simulink model "AutomotiveEMS_2017b"  (R2017b)
settings: Solver=VariableStepAuto  StartTime=0  StopTime=0.1  MaxStep=1e-4  RelTol=1e-3
values from neighbouring files (symbols this model uses):
  iceToAltRotRatio = 2.5    [AutomotiveEMSRoutine.m]    (also in ControlComparisonRoutine.m; Main.m)
  T_s = 1.0e-6    (= 1e-06)    [AutomotiveEMSRoutine.m]    (also in ControlComparisonRoutine.m; HybridMPPTRoutine.m; LundellAlternatorACRoutine.m; LundellAlternatorDCRoutine.m)
undefined symbols (not defined in the file or in its folder): alternator, sigbuilder_block
libraries: fl_lib x74, nesl_utility x72, elec_lib x35, powerlib_meascontrol x2
(part 1 of 2)
settings Model: Creator=gabrielrodrigues  LastModifiedBy=gabrielrodrigues
settings CodeAppCC: StateflowObjectComments=on
settings SimscapeCC: SimscapeNormalizeSystem=off

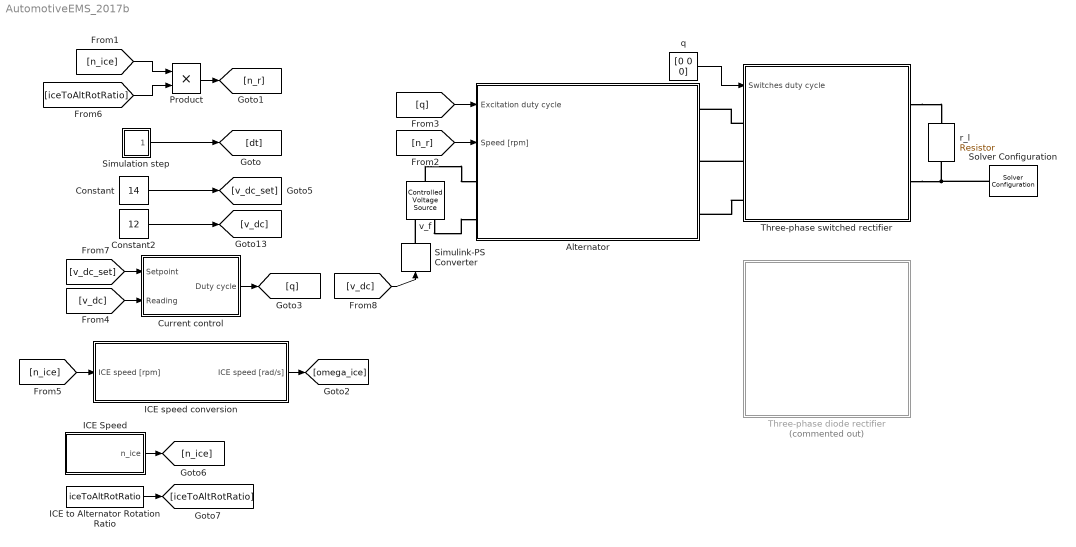
== system AutomotiveEMS_2017b ==
  Alternator : Subsystem
  Constant : Constant  Value=14
  Constant2 : Constant  Value=12
  Current control : Subsystem
  ICE Speed : Subsystem  Tag=STV Subsys  LoadFcn=sigbuilder_block('load');  StartFcn=sigbuilder_block('start');  StopFcn=sigbuilder_block('stop');  ClipboardFcn=sigbuilder_block('clipboard');  mask(Sigbuilder block){tuvar=[0:10]}
      mask help: Simulink:masks:SigbuilderBlock_MD
      mask init:
      | if ~strcmp(get_param(bdroot(gcbh),'SimulationStatus'),'stopped') tuvar = sigbuilder_block('maskInit'); end
      settings: CopyFcn=sigbuilder_block('copy');  DeleteFcn=sigbuilder_block('delete');  ModelCloseFcn=sigbuilder_block('modelClose');  PreSaveFcn=sigbuilder_block('preSave');  PauseFcn=sigbuilder_block('pause');  ContinueFcn=sigbuilder_block('continue');  NameChangeFcn=sigbuilder_block('namechange');  OpenFcn=sigbuilder_block('open',[433.5 195.75 558 399.75 ]);  CloseFcn=sigbuilder_block('close');
      mask Display: plot(0, 0, 100, 100,[2, 2, 32, 32, 2], [68, 8, 8, 68, 68],[32, 2], [38, 38], [32, 19, 2],[53, 60, 44], [32, 17, 17, 2],[16, 16, 31, 31]);txt = getActiveGroup(gcbh);text(2, 100, txt,'verticalAlignment', 'top');
  ICE speed conversion : Subsystem
  ICE to Alternator Rotation Ratio : Constant  Value=iceToAltRotRatio
  Product : Product
  Simulation step : Subsystem
  Simulink-PS Converter : nesl_utility/Simulink-PS Converter  PhysicalDomain=network_engine_domain  SubClassName=ps_input  LeftPortType=input  RightPortType=output  PseudoPeriodic=off  Frequencies=[]  NoiseDistribution=none  NoiseParameters=[]  Unit=1  AffineConversion=off  FilteringAndDerivatives=provide  SimscapeFilterOrder=1  InputFilterTimeConstant=0.001  UdotUserProvided=0
  Solver Configuration : nesl_utility/Solver Configuration  PhysicalDomain=network_engine_domain  SubClassName=solver  LeftPortType=input  RightPortType=generic  Tones=[]  Harmonics=[]  SimulateNoise=off  Profile=off  UseLocalSampling=off  EnableSwitchedLinearOptims=on  FrequencyDomain=off  UseCCode=off  RelTol=0.001  AbsTol=1e-06  MinStep=1e-09  ToWorkspace=off  RevertToSquareIcSolve=off  NumHomotopyIterations=100  PhasorMode=off  PhasorModeNumHarmonics=1  DoDC=off  ResidualTolerance=1e-09  UseLocalSolver=off  LocalSolverChoice=NE_BACKWARD_EULER_ADVANCER  LocalSolverSampleTime=0.001  DoFixedCost=off  MaxNonlinIter=3  MaxModeIter=2  LinearAlgebra=Sparse  EquationFormulation=NE_TIME_EF  DelaysMemoryBudget=1024  AutomaticFiltering=on  FilteringTimeConstant=0.001
  Three-phase diode rectifier : Subsystem  Commented=on
  Three-phase switched rectifier : Subsystem
  q : Constant  Value=[0 0 0]
  r_l : elec_lib/Passive Devices/Resistor  R=1e+3 Ohm  R_tol=5  enable_R_tol=0  tol_distribution=1  nSigma=4  enable_operating_limits=0  operating_limit_action=2  max_working_voltage=100 V  power_rating=1 W  enable_faults=0  fault_action=1  R_faulted=inf Ohm  enable_temporal_fault=0  t_fault=1 s  enable_behavioral_fault=0  max_permissible_current=1 A  t_fail_on_current=1 s  noise_mode=0  sample_time=1e-3 s  repeatability=1  auto_seed=3922919431  user_seed=0  Tdevice=25 degC  alpha=3.93e-3 1/K  Tmeas=25 degC  thermal_mass=100 J/K  power_derating_T1=70 degC  power_derating_T2=155 degC  operating_temperature_range_vec=[-50, 150] degC  temperature_specify=off  temperature_priority=High  temperature=298.15 K  temperature_nominal_specify=off  temperature_nominal_unit=K  temperature_nominal_value=1
  v_f : fl_lib/Electrical/Electrical Sources/Controlled Voltage Source
  wires:
  [iceToAltRotRatio] -> Product/2
  [n_ice] -> Product/1
  Product/1 -> [n_r]
  Simulation step/1(step) -> [dt]
  ICE speed conversion/1(ICE speed [rad/s]) -> [omega_ice]
  Constant/1 -> [v_dc_set]
  [n_ice] -> ICE speed conversion/1(ICE speed [rpm])
  ICE to Alternator Rotation Ratio/1 -> [iceToAltRotRatio]
  Constant2/1 -> [v_dc]
  ICE Speed/1(n_ice) -> [n_ice]
  [n_r] -> Alternator/2(Speed [rpm])
  [q] -> Alternator/1(Excitation duty cycle)
  [v_dc] -> Current control/2(Reading)
  [v_dc_set] -> Current control/1(Setpoint)
  Current control/1(Duty cycle) -> [q]
  [v_dc] -> Simulink-PS Converter/1
  q/1 -> Three-phase switched rectifier/1(Switches duty cycle)
  connections:
  Three-phase switched rectifier/RConn1 -- r_l/LConn1
  Three-phase switched rectifier/LConn2 -- Alternator/RConn2
  Three-phase switched rectifier/LConn3 -- Alternator/RConn3
  Three-phase switched rectifier/LConn1 -- Alternator/RConn1
  Solver Configuration/RConn1 -- Three-phase switched rectifier/RConn2 -- r_l/RConn1
  v_f/LConn1 -- Alternator/LConn1
  v_f/RConn2 -- Alternator/LConn2
  Simulink-PS Converter/RConn1 -- v_f/RConn1

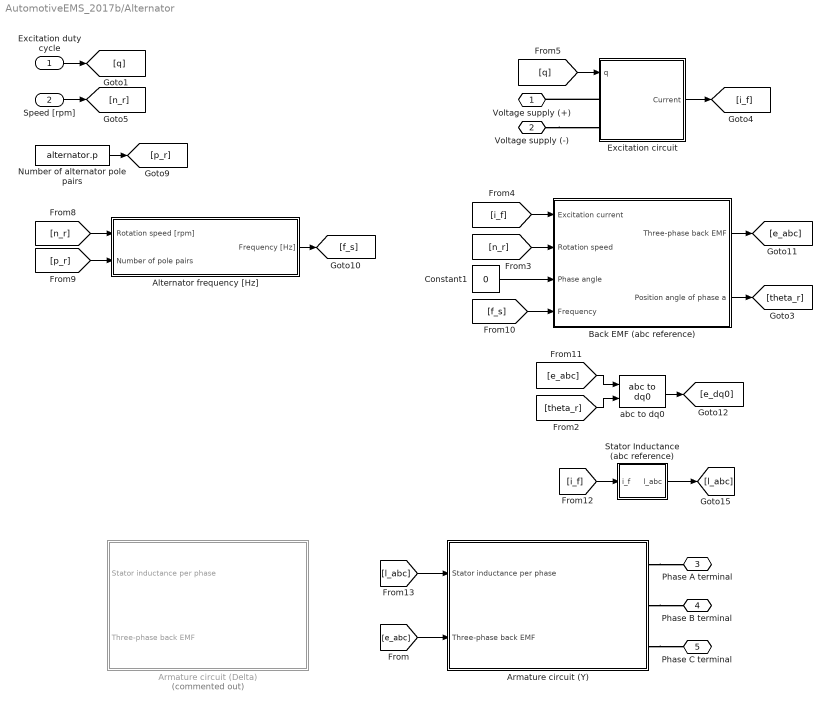
== system AutomotiveEMS_2017b/Alternator ==
  Excitation duty cycle : Inport
  Speed [rpm] : Inport  Port=2
  Alternator frequency [Hz] : Subsystem
  Armature circuit (Delta) : Subsystem  Commented=on
  Armature circuit (Y) : Subsystem
  Back EMF (abc reference) : Subsystem
  Constant1 : Constant  Value=0
  Excitation circuit : Subsystem
  Number of alternator pole pairs : Constant  Value=alternator.p
  Stator Inductance (abc reference) : Subsystem
  abc to dq0 : powerlib_meascontrol/Transformations/abc to dq0  Alignment=90 degrees behind phase A axis
  Voltage supply (+) : PMIOPort  Side=Left
  Voltage supply (-) : PMIOPort  Port=2  Side=Left
  Phase A terminal : PMIOPort  Port=3  Side=Right
  Phase B terminal : PMIOPort  Port=4  Side=Right
  Phase C terminal : PMIOPort  Port=5  Side=Right
  wires:
  Excitation circuit/1(Current) -> [i_f]
  Alternator frequency [Hz]/1(Frequency [Hz]) -> [f_s]
  Number of alternator pole pairs/1 -> [p_r]
  [n_r] -> Alternator frequency [Hz]/1(Rotation speed [rpm])
  [p_r] -> Alternator frequency [Hz]/2(Number of pole pairs)
  [i_f] -> Back EMF (abc reference)/1(Excitation current)
  [n_r] -> Back EMF (abc reference)/2(Rotation speed)
  Constant1/1 -> Back EMF (abc reference)/3(Phase angle)
  [f_s] -> Back EMF (abc reference)/4(Frequency)
  Back EMF (abc reference)/1(Three-phase back EMF) -> [e_abc]
  Back EMF (abc reference)/2(Position angle of phase a) -> [theta_r]
  [e_abc] -> abc to dq0/1
  [theta_r] -> abc to dq0/2
  abc to dq0/1 -> [e_dq0]
  [i_f] -> Stator Inductance (abc reference)/1(i_f)
  Stator Inductance (abc reference)/1(l_abc) -> [l_abc]
  [l_abc] -> Armature circuit (Y)/1(Stator inductance per phase)
  [e_abc] -> Armature circuit (Y)/2(Three-phase back EMF)
  Excitation duty cycle/1 -> [q]
  Speed [rpm]/1 -> [n_r]
  [q] -> Excitation circuit/1(q)
  connections:
  Armature circuit (Y)/RConn1 -- Phase A terminal/RConn1
  Armature circuit (Y)/RConn2 -- Phase B terminal/RConn1
  Armature circuit (Y)/RConn3 -- Phase C terminal/RConn1
  Excitation circuit/LConn1 -- Voltage supply (+)/RConn1
  Voltage supply (-)/RConn1 -- Excitation circuit/LConn2

== system AutomotiveEMS_2017b/Current control ==
  Setpoint : Inport
  Reading : Inport  Port=2
  Fcn : Fcn  Expr=u > 0
  Scope : Scope
  Sum : Sum  Inputs=+-
  Duty cycle : Outport
  wires:
  Fcn/1 -> Duty cycle/1, Scope/1
  Reading/1 -> Sum/2
  Setpoint/1 -> Sum/1
  Sum/1 -> Fcn/1

== system AutomotiveEMS_2017b/ICE Speed ==
  Demux : Demux  Tag=STV Demux  Outputs=1
  FromWs : FromWorkspace  Tag=STV FromWs  VariableName=tuvar  SampleTime=0
      SigBuilderData=|
      | common.afterFinalStr = 'Extrapolate'
      | common.sampleTime = 0
      | dataSet.timeRange = [0 10]
      | dataSet.name = 'Group 1'
      | sbobj.Groups.Name = 'Group 1'
      | sbobj.Groups.Signals.Name = 'n_ice'
      | sbobj.Groups.Signals.XData = [0 2 7 10]
      | sbobj.Groups.Signals.YData = [0 900 900 0]
  n_ice : Outport  Tag=STV Outport
  wires:
  FromWs/1 -> Demux/1
  Demux/1 -> n_ice/1

== system AutomotiveEMS_2017b/ICE speed conversion ==
  ICE speed [rpm] : Inport
  Gain : Gain  Gain=2*pi/60
  ICE speed [rad/s] : Outport
  wires:
  ICE speed [rpm]/1 -> Gain/1
  Gain/1 -> ICE speed [rad/s]/1

== system AutomotiveEMS_2017b/Simulation step ==
  Clock : Clock
  Memory : Memory
  Sum : Sum  Inputs=|-+
  step : Outport
  wires:
  Clock/1 -> Sum/2, Memory/1
  Memory/1 -> Sum/1
  Sum/1 -> step/1

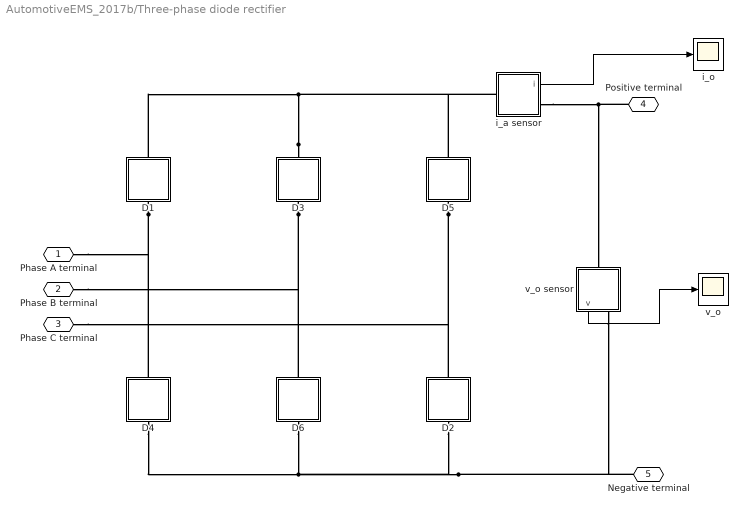
== system AutomotiveEMS_2017b/Three-phase diode rectifier ==
  D1 : Subsystem
  D2 : Subsystem
  D3 : Subsystem
  D4 : Subsystem
  D5 : Subsystem
  D6 : Subsystem
  i_a sensor : Subsystem
  i_o : Scope
  v_o : Scope
  v_o sensor : Subsystem
  Phase A terminal : PMIOPort  Side=Left
  Phase B terminal : PMIOPort  Port=2  Side=Left
  Phase C terminal : PMIOPort  Port=3  Side=Left
  Positive terminal : PMIOPort  Port=4  Side=Right
  Negative terminal : PMIOPort  Port=5  Side=Right
  wires:
  v_o sensor/1(v) -> v_o/1
  i_a sensor/1(i) -> i_o/1
  connections:
  D3/LConn1 -- Phase B terminal/RConn1 -- D6/RConn1
  D1/LConn1 -- Phase A terminal/RConn1 -- D4/RConn1
  D3/RConn1 -- D1/RConn1 -- D5/RConn1 -- i_a sensor/LConn1
  D4/LConn1 -- D6/LConn1 -- D2/LConn1 -- v_o sensor/RConn1 -- Negative terminal/RConn1
  i_a sensor/RConn1 -- Positive terminal/RConn1 -- v_o sensor/LConn1
  D5/LConn1 -- Phase C terminal/RConn1 -- D2/RConn1

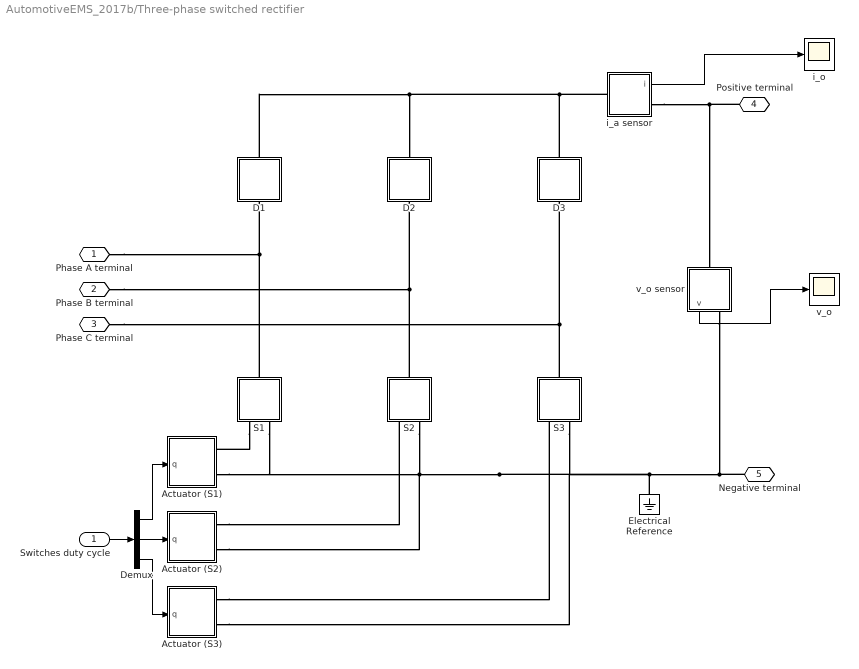
== system AutomotiveEMS_2017b/Three-phase switched rectifier ==
  Switches duty cycle : Inport
  Actuator (S1) : Subsystem
  Actuator (S2) : Subsystem
  Actuator (S3) : Subsystem
  D1 : Subsystem
  D2 : Subsystem
  D3 : Subsystem
  Demux : Demux  Outputs=3
  Electrical Reference : fl_lib/Electrical/Electrical Elements/Electrical Reference
  S1 : Subsystem
  S2 : Subsystem
  S3 : Subsystem
  i_a sensor : Subsystem
  i_o : Scope
  v_o : Scope
  v_o sensor : Subsystem
  Phase A terminal : PMIOPort  Side=Left
  Phase B terminal : PMIOPort  Port=2  Side=Left
  Phase C terminal : PMIOPort  Port=3  Side=Left
  Positive terminal : PMIOPort  Port=4  Side=Right
  Negative terminal : PMIOPort  Port=5  Side=Right
  wires:
  v_o sensor/1(v) -> v_o/1
  i_a sensor/1(i) -> i_o/1
  Demux/2 -> Actuator (S2)/1(q)
  Demux/1 -> Actuator (S1)/1(q)
  Demux/3 -> Actuator (S3)/1(q)
  Switches duty cycle/1 -> Demux/1
  connections:
  Phase B terminal/RConn1 -- S2/RConn1 -- D2/LConn1
  Phase A terminal/RConn1 -- S1/RConn1 -- D1/LConn1
  i_a sensor/LConn1 -- D2/RConn1 -- D1/RConn1 -- D3/RConn1
  v_o sensor/RConn1 -- Electrical Reference/LConn1 -- Actuator (S3)/RConn2 -- S3/LConn2 -- Actuator (S2)/RConn2 -- S1/LConn2 -- Actuator (S1)/RConn2 -- S2/LConn2 -- Negative terminal/RConn1
  Positive terminal/RConn1 -- i_a sensor/RConn1 -- v_o sensor/LConn1
  Phase C terminal/RConn1 -- S3/RConn1 -- D3/LConn1
  S1/LConn1 -- Actuator (S1)/RConn1
  Actuator (S2)/RConn1 -- S2/LConn1
  Actuator (S3)/RConn1 -- S3/LConn1

== system AutomotiveEMS_2017b/Alternator/Alternator frequency [Hz] ==
  Rotation speed [rpm] : Inport
  Number of pole pairs : Inport  Port=2
  Gain : Gain  Gain=1/60
  Product1 : Product
  Frequency [Hz] : Outport
  wires:
  Rotation speed [rpm]/1 -> Product1/1
  Gain/1 -> Frequency [Hz]/1
  Product1/1 -> Gain/1
  Number of pole pairs/1 -> Product1/2

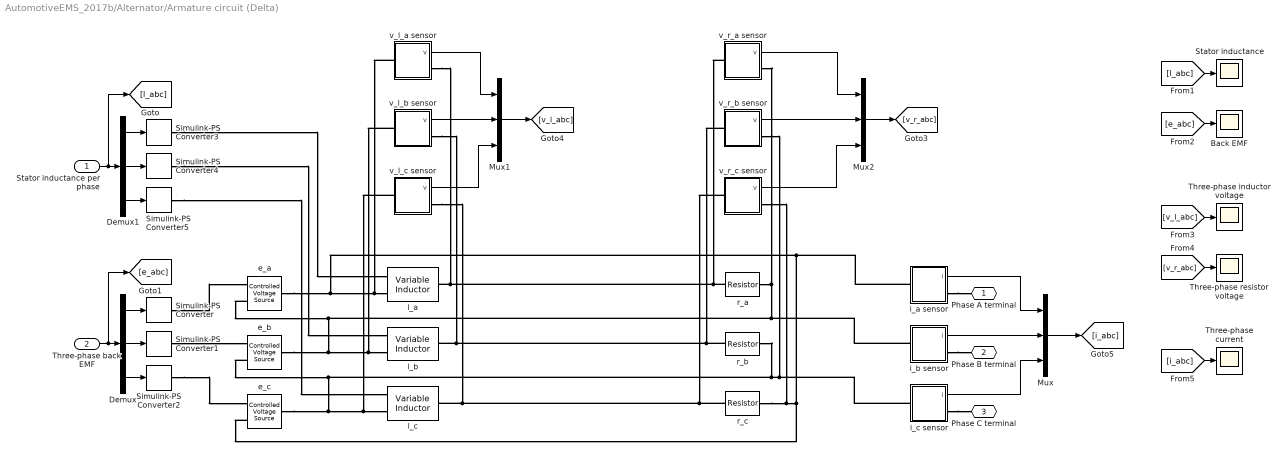
== system AutomotiveEMS_2017b/Alternator/Armature circuit (Delta) ==
  Stator inductance per phase : Inport
  Three-phase back EMF : Inport  Port=2
  Back EMF : Scope
  Demux : Demux  Outputs=3
  Demux1 : Demux  Outputs=3
  Mux : Mux  Inputs=3
  Mux1 : Mux  Inputs=3
  Mux2 : Mux  Inputs=3
  Simulink-PS Converter : nesl_utility/Simulink-PS Converter  PhysicalDomain=network_engine_domain  SubClassName=ps_input  LeftPortType=input  RightPortType=output  PseudoPeriodic=off  Frequencies=[]  NoiseDistribution=none  NoiseParameters=[]  Unit=V  AffineConversion=on  FilteringAndDerivatives=filter  SimscapeFilterOrder=2  InputFilterTimeConstant=0.001  UdotUserProvided=0
  Simulink-PS Converter1 : nesl_utility/Simulink-PS Converter  PhysicalDomain=network_engine_domain  SubClassName=ps_input  LeftPortType=input  RightPortType=output  PseudoPeriodic=off  Frequencies=[]  NoiseDistribution=none  NoiseParameters=[]  Unit=V  AffineConversion=off  FilteringAndDerivatives=filter  SimscapeFilterOrder=2  InputFilterTimeConstant=0.001  UdotUserProvided=0
  Simulink-PS Converter2 : nesl_utility/Simulink-PS Converter  PhysicalDomain=network_engine_domain  SubClassName=ps_input  LeftPortType=input  RightPortType=output  PseudoPeriodic=off  Frequencies=[]  NoiseDistribution=none  NoiseParameters=[]  Unit=V  AffineConversion=off  FilteringAndDerivatives=filter  SimscapeFilterOrder=2  InputFilterTimeConstant=0.001  UdotUserProvided=0
  Simulink-PS Converter3 : nesl_utility/Simulink-PS Converter  PhysicalDomain=network_engine_domain  SubClassName=ps_input  LeftPortType=input  RightPortType=output  PseudoPeriodic=off  Frequencies=[]  NoiseDistribution=none  NoiseParameters=[]  Unit=1  AffineConversion=off  FilteringAndDerivatives=provide  SimscapeFilterOrder=1  InputFilterTimeConstant=0.001  UdotUserProvided=0
  Simulink-PS Converter4 : nesl_utility/Simulink-PS Converter  PhysicalDomain=network_engine_domain  SubClassName=ps_input  LeftPortType=input  RightPortType=output  PseudoPeriodic=off  Frequencies=[]  NoiseDistribution=none  NoiseParameters=[]  Unit=1  AffineConversion=off  FilteringAndDerivatives=provide  SimscapeFilterOrder=1  InputFilterTimeConstant=0.001  UdotUserProvided=0
  Simulink-PS Converter5 : nesl_utility/Simulink-PS Converter  PhysicalDomain=network_engine_domain  SubClassName=ps_input  LeftPortType=input  RightPortType=output  PseudoPeriodic=off  Frequencies=[]  NoiseDistribution=none  NoiseParameters=[]  Unit=1  AffineConversion=off  FilteringAndDerivatives=provide  SimscapeFilterOrder=1  InputFilterTimeConstant=0.001  UdotUserProvided=0
  Stator inductance : Scope
  Three-phase current : Scope
  Three-phase inductor voltage : Scope
  Three-phase resistor voltage : Scope
  e_a : fl_lib/Electrical/Electrical Sources/Controlled Voltage Source
  e_b : fl_lib/Electrical/Electrical Sources/Controlled Voltage Source
  e_c : fl_lib/Electrical/Electrical Sources/Controlled Voltage Source
  i_a sensor : Subsystem
  i_b sensor : Subsystem
  i_c sensor : Subsystem
  l_a : elec_lib/Passive Devices/Variable Inductor  prm=1  Lmin=1e-6 H  g=1e-9 1/Ohm  i0=0 A  phi0=0 Wb
      settings: SourceProductName=Simscape Electronics  SourceProductBaseCode=SN
  l_b : elec_lib/Passive Devices/Variable Inductor  prm=1  Lmin=1e-6 H  g=1e-9 1/Ohm  i0=0 A  phi0=0 Wb
      settings: SourceProductName=Simscape Electronics  SourceProductBaseCode=SN
  l_c : elec_lib/Passive Devices/Variable Inductor  prm=1  Lmin=1e-6 H  g=1e-9 1/Ohm  i0=0 A  phi0=0 Wb
      settings: SourceProductName=Simscape Electronics  SourceProductBaseCode=SN
  r_a : elec_lib/Passive Devices/Resistor  R=alternator.stator.r Ohm  R_tol=5  enable_R_tol=0  tol_distribution=1  nSigma=4  enable_operating_limits=0  operating_limit_action=2  max_working_voltage=100 V  power_rating=1 W  enable_faults=0  fault_action=1  R_faulted=inf Ohm  enable_temporal_fault=0  t_fault=1 s  enable_behavioral_fault=0  max_permissible_current=1 A  t_fail_on_current=1 s  noise_mode=0  sample_time=1e-3 s  repeatability=1  auto_seed=2033606855  user_seed=0  Tdevice=25 degC  alpha=3.93e-3 1/K  Tmeas=25 degC  thermal_mass=100 J/K  power_derating_T1=70 degC  power_derating_T2=155 degC  operating_temperature_range_vec=[-50, 150] degC  temperature_specify=off  temperature_priority=High  temperature=298.15 K  temperature_nominal_specify=off  temperature_nominal_unit=K  temperature_nominal_value=1
  r_b : elec_lib/Passive Devices/Resistor  R=alternator.stator.r Ohm  R_tol=5  enable_R_tol=0  tol_distribution=1  nSigma=4  enable_operating_limits=0  operating_limit_action=2  max_working_voltage=100 V  power_rating=1 W  enable_faults=0  fault_action=1  R_faulted=inf Ohm  enable_temporal_fault=0  t_fault=1 s  enable_behavioral_fault=0  max_permissible_current=1 A  t_fail_on_current=1 s  noise_mode=0  sample_time=1e-3 s  repeatability=1  auto_seed=655932562  user_seed=0  Tdevice=25 degC  alpha=3.93e-3 1/K  Tmeas=25 degC  thermal_mass=100 J/K  power_derating_T1=70 degC  power_derating_T2=155 degC  operating_temperature_range_vec=[-50, 150] degC  temperature_specify=off  temperature_priority=High  temperature=298.15 K  temperature_nominal_specify=off  temperature_nominal_unit=K  temperature_nominal_value=1
  r_c : elec_lib/Passive Devices/Resistor  R=alternator.stator.r Ohm  R_tol=5  enable_R_tol=0  tol_distribution=1  nSigma=4  enable_operating_limits=0  operating_limit_action=2  max_working_voltage=100 V  power_rating=1 W  enable_faults=0  fault_action=1  R_faulted=inf Ohm  enable_temporal_fault=0  t_fault=1 s  enable_behavioral_fault=0  max_permissible_current=1 A  t_fail_on_current=1 s  noise_mode=0  sample_time=1e-3 s  repeatability=1  auto_seed=1465119031  user_seed=0  Tdevice=25 degC  alpha=3.93e-3 1/K  Tmeas=25 degC  thermal_mass=100 J/K  power_derating_T1=70 degC  power_derating_T2=155 degC  operating_temperature_range_vec=[-50, 150] degC  temperature_specify=off  temperature_priority=High  temperature=298.15 K  temperature_nominal_specify=off  temperature_nominal_unit=K  temperature_nominal_value=1
  v_l_a sensor : Subsystem
  v_l_b sensor : Subsystem
  v_l_c sensor : Subsystem
  v_r_a sensor : Subsystem
  v_r_b sensor : Subsystem
  v_r_c sensor : Subsystem
  Phase A terminal : PMIOPort  Side=Right
  Phase B terminal : PMIOPort  Port=2  Side=Right
  Phase C terminal : PMIOPort  Port=3  Side=Right
  wires:
  Three-phase back EMF/1 -> [e_abc], Demux/1
  Demux/1 -> Simulink-PS Converter/1
  Demux/2 -> Simulink-PS Converter1/1
  Demux/3 -> Simulink-PS Converter2/1
  Demux1/1 -> Simulink-PS Converter3/1
  Demux1/3 -> Simulink-PS Converter5/1
  Demux1/2 -> Simulink-PS Converter4/1
  Stator inductance per phase/1 -> [l_abc], Demux1/1
  i_a sensor/1(i) -> Mux/1
  i_b sensor/1(i) -> Mux/2
  i_c sensor/1(i) -> Mux/3
  Mux/1 -> [i_abc]
  Mux1/1 -> [v_l_abc]
  v_l_a sensor/1(v) -> Mux1/1
  v_l_c sensor/1(v) -> Mux1/3
  v_l_b sensor/1(v) -> Mux1/2
  Mux2/1 -> [v_r_abc]
  v_r_a sensor/1(v) -> Mux2/1
  v_r_c sensor/1(v) -> Mux2/3
  v_r_b sensor/1(v) -> Mux2/2
  [l_abc] -> Stator inductance/1
  [e_abc] -> Back EMF/1
  [v_l_abc] -> Three-phase inductor voltage/1
  [v_r_abc] -> Three-phase resistor voltage/1
  [i_abc] -> Three-phase current/1
  connections:
  i_a sensor/RConn1 -- Phase A terminal/RConn1
  Simulink-PS Converter/RConn1 -- e_a/RConn1
  Simulink-PS Converter1/RConn1 -- e_b/RConn1
  Simulink-PS Converter2/RConn1 -- e_c/RConn1
  r_c/LConn1 -- v_l_c sensor/RConn1 -- l_c/RConn1 -- v_r_c sensor/LConn1
  r_b/LConn1 -- v_l_b sensor/RConn1 -- l_b/RConn1 -- v_r_b sensor/LConn1
  r_a/LConn1 -- v_l_a sensor/RConn1 -- l_a/RConn1 -- v_r_a sensor/LConn1
  i_c sensor/RConn1 -- Phase C terminal/RConn1
  i_b sensor/RConn1 -- Phase B terminal/RConn1
  Simulink-PS Converter5/RConn1 -- l_c/LConn1
  Simulink-PS Converter4/RConn1 -- l_b/LConn1
  Simulink-PS Converter3/RConn1 -- l_a/LConn1
  v_r_a sensor/RConn1 -- i_b sensor/LConn1 -- e_b/LConn1 -- v_l_b sensor/LConn1 -- l_b/LConn2 -- e_a/RConn2 -- r_a/RConn1
  i_c sensor/LConn1 -- r_b/RConn1 -- e_b/RConn2 -- e_c/LConn1 -- v_l_c sensor/LConn1 -- l_c/LConn2 -- v_r_b sensor/RConn1
  r_c/RConn1 -- e_c/RConn2 -- i_a sensor/LConn1 -- e_a/LConn1 -- v_l_a sensor/LConn1 -- l_a/LConn2 -- v_r_c sensor/RConn1

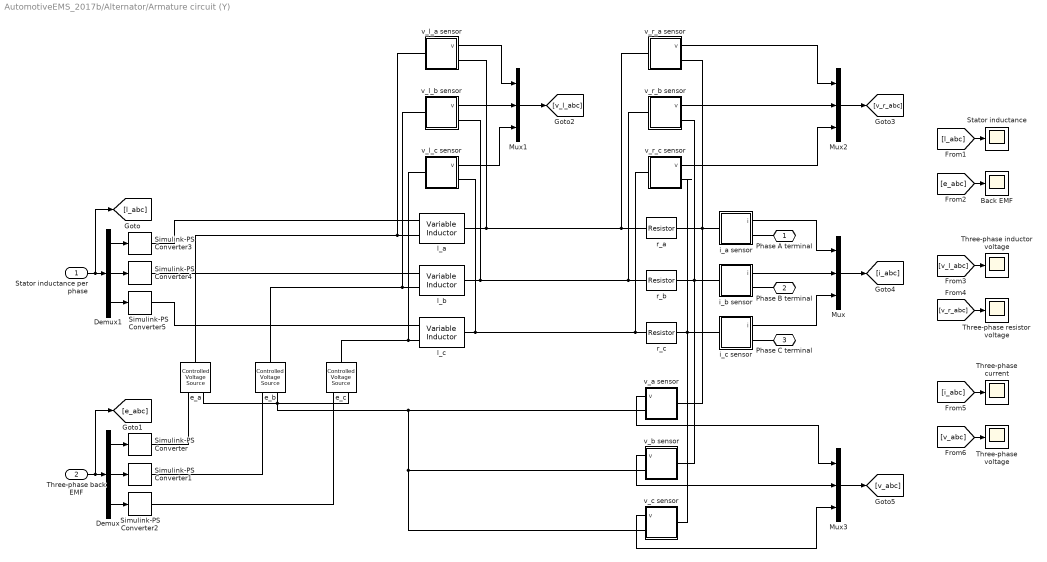
== system AutomotiveEMS_2017b/Alternator/Armature circuit (Y) ==
  Stator inductance per phase : Inport
  Three-phase back EMF : Inport  Port=2
  Back EMF : Scope
  Demux : Demux  Outputs=3
  Demux1 : Demux  Outputs=3
  Mux{,1..3} (4 alike) : Mux  Inputs=3
  Simulink-PS Converter{,1..5} (6 alike) : nesl_utility/Simulink-PS Converter  PhysicalDomain=network_engine_domain  SubClassName=ps_input  LeftPortType=input  RightPortType=output  PseudoPeriodic=off  Frequencies=[]  NoiseDistribution=none  NoiseParameters=[]  Unit=1  AffineConversion=off  FilteringAndDerivatives=provide  SimscapeFilterOrder=1  InputFilterTimeConstant=0.001  UdotUserProvided=0
  Stator inductance : Scope
  Three-phase current : Scope
  Three-phase inductor voltage : Scope
  Three-phase resistor voltage : Scope
  Three-phase voltage : Scope
  e_a : fl_lib/Electrical/Electrical Sources/Controlled Voltage Source
  e_b : fl_lib/Electrical/Electrical Sources/Controlled Voltage Source
  e_c : fl_lib/Electrical/Electrical Sources/Controlled Voltage Source
  i_a sensor : Subsystem
  i_b sensor : Subsystem
  i_c sensor : Subsystem
  l_a : elec_lib/Passive Devices/Variable Inductor  prm=1  Lmin=1e-6 H  g=1e-9 1/Ohm  i0=0 A  phi0=0 Wb
      settings: SourceProductName=Simscape Electronics  SourceProductBaseCode=SN
  l_b : elec_lib/Passive Devices/Variable Inductor  prm=1  Lmin=1e-6 H  g=1e-9 1/Ohm  i0=0 A  phi0=0 Wb
      settings: SourceProductName=Simscape Electronics  SourceProductBaseCode=SN
  l_c : elec_lib/Passive Devices/Variable Inductor  prm=1  Lmin=1e-6 H  g=1e-9 1/Ohm  i0=0 A  phi0=0 Wb
      settings: SourceProductName=Simscape Electronics  SourceProductBaseCode=SN
  r_a : elec_lib/Passive Devices/Resistor  R=alternator.stator.r Ohm  R_tol=5  enable_R_tol=0  tol_distribution=1  nSigma=4  enable_operating_limits=0  operating_limit_action=2  max_working_voltage=100 V  power_rating=1 W  enable_faults=0  fault_action=1  R_faulted=inf Ohm  enable_temporal_fault=0  t_fault=1 s  enable_behavioral_fault=0  max_permissible_current=1 A  t_fail_on_current=1 s  noise_mode=0  sample_time=1e-3 s  repeatability=1  auto_seed=153599770  user_seed=0  Tdevice=25 degC  alpha=3.93e-3 1/K  Tmeas=25 degC  thermal_mass=100 J/K  power_derating_T1=70 degC  power_derating_T2=155 degC  operating_temperature_range_vec=[-50, 150] degC  temperature_specify=off  temperature_priority=High  temperature=298.15 K  temperature_nominal_specify=off  temperature_nominal_unit=K  temperature_nominal_value=1
  r_b : elec_lib/Passive Devices/Resistor  R=alternator.stator.r Ohm  R_tol=5  enable_R_tol=0  tol_distribution=1  nSigma=4  enable_operating_limits=0  operating_limit_action=2  max_working_voltage=100 V  power_rating=1 W  enable_faults=0  fault_action=1  R_faulted=inf Ohm  enable_temporal_fault=0  t_fault=1 s  enable_behavioral_fault=0  max_permissible_current=1 A  t_fail_on_current=1 s  noise_mode=0  sample_time=1e-3 s  repeatability=1  auto_seed=755374864  user_seed=0  Tdevice=25 degC  alpha=3.93e-3 1/K  Tmeas=25 degC  thermal_mass=100 J/K  power_derating_T1=70 degC  power_derating_T2=155 degC  operating_temperature_range_vec=[-50, 150] degC  temperature_specify=off  temperature_priority=High  temperature=298.15 K  temperature_nominal_specify=off  temperature_nominal_unit=K  temperature_nominal_value=1
  r_c : elec_lib/Passive Devices/Resistor  R=alternator.stator.r Ohm  R_tol=5  enable_R_tol=0  tol_distribution=1  nSigma=4  enable_operating_limits=0  operating_limit_action=2  max_working_voltage=100 V  power_rating=1 W  enable_faults=0  fault_action=1  R_faulted=inf Ohm  enable_temporal_fault=0  t_fault=1 s  enable_behavioral_fault=0  max_permissible_current=1 A  t_fail_on_current=1 s  noise_mode=0  sample_time=1e-3 s  repeatability=1  auto_seed=3099927149  user_seed=0  Tdevice=25 degC  alpha=3.93e-3 1/K  Tmeas=25 degC  thermal_mass=100 J/K  power_derating_T1=70 degC  power_derating_T2=155 degC  operating_temperature_range_vec=[-50, 150] degC  temperature_specify=off  temperature_priority=High  temperature=298.15 K  temperature_nominal_specify=off  temperature_nominal_unit=K  temperature_nominal_value=1
  v_a sensor : Subsystem
  v_b sensor : Subsystem
  v_c sensor : Subsystem
  v_l_a sensor : Subsystem
  v_l_b sensor : Subsystem
  v_l_c sensor : Subsystem
  v_r_a sensor : Subsystem
  v_r_b sensor : Subsystem
  v_r_c sensor : Subsystem
  Phase A terminal : PMIOPort  Side=Right
  Phase B terminal : PMIOPort  Port=2  Side=Right
  Phase C terminal : PMIOPort  Port=3  Side=Right
  wires:
  Three-phase back EMF/1 -> [e_abc], Demux/1
  Demux/1 -> Simulink-PS Converter/1
  Demux/2 -> Simulink-PS Converter1/1
  Demux/3 -> Simulink-PS Converter2/1
  Demux1/1 -> Simulink-PS Converter3/1
  Demux1/3 -> Simulink-PS Converter5/1
  Demux1/2 -> Simulink-PS Converter4/1
  Stator inductance per phase/1 -> [l_abc], Demux1/1
  i_a sensor/1(i) -> Mux/1
  i_b sensor/1(i) -> Mux/2
  i_c sensor/1(i) -> Mux/3
  Mux/1 -> [i_abc]
  v_r_b sensor/1(v) -> Mux2/2
  Mux2/1 -> [v_r_abc]
  Mux3/1 -> [v_abc]
  v_b sensor/1(v) -> Mux3/2
  v_c sensor/1(v) -> Mux3/3
  v_a sensor/1(v) -> Mux3/1
  v_l_b sensor/1(v) -> Mux1/2
  v_l_c sensor/1(v) -> Mux1/3
  v_l_a sensor/1(v) -> Mux1/1
  v_r_c sensor/1(v) -> Mux2/3
  v_r_a sensor/1(v) -> Mux2/1
  Mux1/1 -> [v_l_abc]
  [i_abc] -> Three-phase current/1
  [v_abc] -> Three-phase voltage/1
  [v_r_abc] -> Three-phase resistor voltage/1
  [e_abc] -> Back EMF/1
  [l_abc] -> Stator inductance/1
  [v_l_abc] -> Three-phase inductor voltage/1
  connections:
  i_a sensor/RConn1 -- Phase A terminal/RConn1
  Simulink-PS Converter/RConn1 -- e_a/RConn1
  Simulink-PS Converter1/RConn1 -- e_b/RConn1
  Simulink-PS Converter2/RConn1 -- e_c/RConn1
  e_a/RConn2 -- v_a sensor/RConn1 -- v_b sensor/RConn1 -- v_c sensor/RConn1 -- e_c/RConn2 -- e_b/RConn2
  e_c/LConn1 -- v_l_c sensor/LConn1 -- l_c/LConn2
  e_b/LConn1 -- v_l_b sensor/LConn1 -- l_b/LConn2
  e_a/LConn1 -- v_l_a sensor/LConn1 -- l_a/LConn2
  r_c/LConn1 -- v_r_c sensor/LConn1 -- v_l_c sensor/RConn1 -- l_c/RConn1
  r_b/LConn1 -- v_r_b sensor/LConn1 -- v_l_b sensor/RConn1 -- l_b/RConn1
  r_a/LConn1 -- v_r_a sensor/LConn1 -- v_l_a sensor/RConn1 -- l_a/RConn1
  Simulink-PS Converter4/RConn1 -- l_b/LConn1
  Simulink-PS Converter5/RConn1 -- l_c/LConn1
  Simulink-PS Converter3/RConn1 -- l_a/LConn1
  i_a sensor/LConn1 -- v_a sensor/LConn1 -- v_r_a sensor/RConn1 -- r_a/RConn1
  i_c sensor/RConn1 -- Phase C terminal/RConn1
  i_b sensor/RConn1 -- Phase B terminal/RConn1
  i_c sensor/LConn1 -- v_c sensor/LConn1 -- v_r_c sensor/RConn1 -- r_c/RConn1
  r_b/RConn1 -- v_b sensor/LConn1 -- v_r_b sensor/RConn1 -- i_b sensor/LConn1

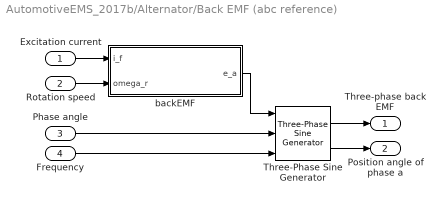
== system AutomotiveEMS_2017b/Alternator/Back EMF (abc reference) ==
  Excitation current : Inport
  Rotation speed : Inport  Port=2
  Phase angle : Inport  Port=3
  Frequency : Inport  Port=4
  Three-Phase Sine Generator : powerlib_meascontrol/Pulse & Signal Generators/Three-Phase Sine Generator  Ts=T_s
      settings: SourceProductName=Simscape Power Systems  SourceProductBaseCode=PS
  backEMF : MATLAB Function  TreatAsAtomicUnit=on
  Three-phase back EMF : Outport
  Position angle of phase a : Outport  Port=2
  wires:
  Three-Phase Sine Generator/1 -> Three-phase back EMF/1
  Phase angle/1 -> Three-Phase Sine Generator/2
  Excitation current/1 -> backEMF/1(i_f)
  Rotation speed/1 -> backEMF/2(omega_r)
  Frequency/1 -> Three-Phase Sine Generator/3
  Three-Phase Sine Generator/2 -> Position angle of phase a/1
  backEMF/1(e_a) -> Three-Phase Sine Generator/1

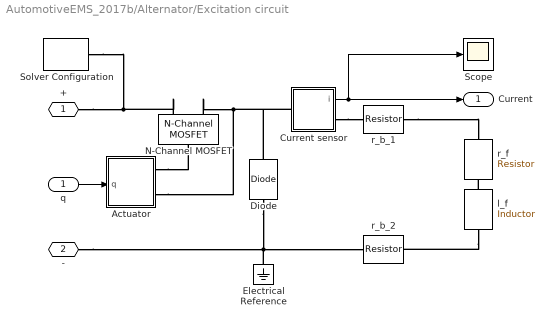
== system AutomotiveEMS_2017b/Alternator/Excitation circuit ==
  q : Inport
  Actuator : Subsystem
  Current sensor : Subsystem
  Diode : elec_lib/Semiconductor Devices/Diode  ModelType=1  Vf=0.5 V  Ron=0.3 Ohm  Goff=1e-8 S  Rz=0.3 Ohm  Vz=50 V  C_PWL=5 pF  prmExp=1  I12=[0.0137, 0.545] A  V12=[0.6, 0.7] V  I1=0.0137 A  V1=0.6 V  IS=1e-12 A  ec=1  RS=0.01 Ohm  Tmeas=25 degC  BV=inf V  C_param=1  CJ0=5 pF  VJ=1 V  Mgrad=0.5  Vvec=[0.1, 10.0, 100.0] V  Cvec=[3.5, 1.0, 0.4] pF  FC=0.5  Q_param=1  Irrm=-7.15 A  iF=4 A  didt=-750 A/us  trr=115 ns  TT=50 ns  tau=100 ns  T_param=1  IS_T2=1.25e-7 A  I1_T2=0.245 A  V1_T2=0.5 V  Tmeas2=125 degC  EG_param=1  EG=1.11 eV  XTI_param=1  XTI=3  dBVdT=0 V/K  Tdevice=25 degC  i_capacitor_specify=off  i_capacitor_priority=High  i_capacitor=0 A  i_capacitor_nominal_specify=off  i_capacitor_nominal_unit=A  i_capacitor_nominal_value=1  v_capacitor_specify=off  v_capacitor_priority=None  v_capacitor=0 V  v_capacitor_nominal_specify=off  v_capacitor_nominal_unit=V  v_capacitor_nominal_value=1  Rth=[0.0, 10.0] K/W  thermal_mass_parameterization=1  thermal_mass=[0.0, 1.0] J/K  thermal_time_constant=[0.0, 10.0] s  thermal_mass_initial_temperatures=[25.0, 25.0] degC
      settings: SourceProductName=Simscape Electronics  SourceProductBaseCode=SN
  Electrical Reference : fl_lib/Electrical/Electrical Elements/Electrical Reference
  N-Channel MOSFET : elec_lib/Semiconductor Devices/N-Channel MOSFET  parameterization=1  prmDatasheet=1  prmEquCoeff=1  Beta=5 A/V^2  Rds=0.1 Ohm  Id=6 A  Vgs=10 V  Vth=1.7 V  lam=0 1/V  Tmeas=25 degC  RS=1e-4 Ohm  RD=0.01 Ohm  C_param=1  C_GS=270 pF  C_GD=80 pF  C_DS=0 pF  C_iss=350 pF  C_rss=80 pF  C_oss=0 pF  C_GS_vec=[ 270 300 290 280 295 255 ] pF  C_GD_vec=[ 450 400 300 190 95 55 ] pF  C_DS_vec=[ 450 410 390 230 175 115 ] pF  C_iss_vec=[ 720 700 590 470 390 310 ] pF  C_rss_vec=[ 450 400 300 190 95 55 ] pF  C_oss_vec=[ 900 810 690 420 270 170 ] pF  C_Vds_vec=[ 0.1 0.3 1 3 10 30 ] V  V_GS_for_cap_data=0 V  charge_linearity_param=1  C_OX=200 pF  V_C_OX=-0.5 V  IsDiode=0 A  Vbi=0.6 V  n=1  Cj0Diode=0 pF  TT=50e-9 s  dVth_dT=-6 mV/K  Rds_T2=0.037 Ohm  Tmeas2=125 degC  BEXDatasheet=-1.5  BEXEquCoeff=-1.5  etaisDatasheet=3  etaisEquCoeff=3  TdeviceDatasheet=25 degC  TdeviceEquCoeff=25 degC  Rth=[1.0, 10.0] K/W  thermal_mass_parameterization=1  thermal_mass=[1.0, 1.0] J/K  thermal_time_constant=[1.0, 10.0] s  thermal_mass_initial_temperatures=[ 25 25 ] degC  betaref=18 A/V^2  Vfbref=-1.1 V  gamma=3.5 V^0.50000  phib2ref=1 V  thesatref=0.4 1/V  alpha=0  Vp=5e-2 V  thesrref=0 1/V  m=8  Tref=25 degC  Cox=1500 pF  Cgso=100 pF  Cgdo=14 pF  Rsref=2e-3 Ohm  Rdref=0.17 Ohm  Rgref=8.4 Ohm  Isref=5.2e-13 A  Cj0=480 pF  Tprm=1  etabet=1.3  Stvfb=5e-4 V/K  Stphib=-8.5e-4 V/K  etasat=1.04  etasr=0.65  etar=0.95  etais=3  Tsim=25 degC  T0=[25.0, 25.0] degC
      settings: SourceProductName=Simscape Electronics  SourceProductBaseCode=SN
  Scope : Scope
  Solver Configuration : nesl_utility/Solver Configuration  PhysicalDomain=network_engine_domain  SubClassName=solver  LeftPortType=input  RightPortType=generic  Tones=[]  Harmonics=[]  SimulateNoise=off  Profile=off  UseLocalSampling=off  EnableSwitchedLinearOptims=on  FrequencyDomain=off  UseCCode=off  RelTol=0.001  AbsTol=1e-06  MinStep=1e-09  ToWorkspace=off  RevertToSquareIcSolve=off  NumHomotopyIterations=100  PhasorMode=off  PhasorModeNumHarmonics=1  DoDC=off  ResidualTolerance=1e-09  UseLocalSolver=off  LocalSolverChoice=NE_BACKWARD_EULER_ADVANCER  LocalSolverSampleTime=0.001  DoFixedCost=off  MaxNonlinIter=3  MaxModeIter=2  LinearAlgebra=Sparse  EquationFormulation=NE_TIME_EF  DelaysMemoryBudget=1024  AutomaticFiltering=on  FilteringTimeConstant=0.001
  l_f : elec_lib/Passive Devices/Inductor  l=alternator.rotor.l H  L_tol=20  enable_L_tol=0  tol_distribution=1  nSigma=4  r=0 Ohm  g=1e-9 1/Ohm  enable_operating_limits=0  operating_limit_action=2  max_working_current=1 A  power_rating=1 W  enable_faults=0  fault_action=1  lambdaPercent=50  k_faulted=0.9999  turnsShort=0  openCct=0  groundShort=0  groundShortG=0 1/Ohm  tau_fault=1e-3 s  enable_temporal_fault=0  t_fault=1 s  enable_behavioral_fault=0  max_permissible_voltage=100 V  n_fail_on_voltage=1  max_permissible_current=1 A  t_fail_on_current=1 s  i_L_specify=off  i_L_priority=High  i_L=0 A  i_L_nominal_specify=off  i_L_nominal_unit=A  i_L_nominal_value=1
      settings: SourceProductName=Simscape Electronics  SourceProductBaseCode=SN
  r_b_1 : elec_lib/Passive Devices/Resistor  R=alternator.rotor.r_b Ohm  R_tol=5  enable_R_tol=0  tol_distribution=1  nSigma=4  enable_operating_limits=0  operating_limit_action=2  max_working_voltage=100 V  power_rating=1 W  enable_faults=0  fault_action=1  R_faulted=inf Ohm  enable_temporal_fault=0  t_fault=1 s  enable_behavioral_fault=0  max_permissible_current=1 A  t_fail_on_current=1 s  noise_mode=0  sample_time=1e-3 s  repeatability=1  auto_seed=2949086957  user_seed=0  Tdevice=25 degC  alpha=3.93e-3 1/K  Tmeas=25 degC  thermal_mass=100 J/K  power_derating_T1=70 degC  power_derating_T2=155 degC  operating_temperature_range_vec=[-50.0, 150.0] degC  temperature_specify=off  temperature_priority=High  temperature=298.15 K  temperature_nominal_specify=off  temperature_nominal_unit=K  temperature_nominal_value=1
  r_b_2 : elec_lib/Passive Devices/Resistor  R=alternator.rotor.r_b Ohm  R_tol=5  enable_R_tol=0  tol_distribution=1  nSigma=4  enable_operating_limits=0  operating_limit_action=2  max_working_voltage=100 V  power_rating=1 W  enable_faults=0  fault_action=1  R_faulted=inf Ohm  enable_temporal_fault=0  t_fault=1 s  enable_behavioral_fault=0  max_permissible_current=1 A  t_fail_on_current=1 s  noise_mode=0  sample_time=1e-3 s  repeatability=1  auto_seed=3089940144  user_seed=0  Tdevice=25 degC  alpha=3.93e-3 1/K  Tmeas=25 degC  thermal_mass=100 J/K  power_derating_T1=70 degC  power_derating_T2=155 degC  operating_temperature_range_vec=[-50.0, 150.0] degC  temperature_specify=off  temperature_priority=High  temperature=298.15 K  temperature_nominal_specify=off  temperature_nominal_unit=K  temperature_nominal_value=1
  r_f : elec_lib/Passive Devices/Resistor  R=alternator.rotor.r_f Ohm  R_tol=5  enable_R_tol=0  tol_distribution=1  nSigma=4  enable_operating_limits=0  operating_limit_action=2  max_working_voltage=100 V  power_rating=1 W  enable_faults=0  fault_action=1  R_faulted=inf Ohm  enable_temporal_fault=0  t_fault=1 s  enable_behavioral_fault=0  max_permissible_current=1 A  t_fail_on_current=1 s  noise_mode=0  sample_time=1e-3 s  repeatability=1  auto_seed=2791903770  user_seed=0  Tdevice=25 degC  alpha=3.93e-3 1/K  Tmeas=25 degC  thermal_mass=100 J/K  power_derating_T1=70 degC  power_derating_T2=155 degC  operating_temperature_range_vec=[-50.0, 150.0] degC  temperature_specify=off  temperature_priority=High  temperature=298.15 K  temperature_nominal_specify=off  temperature_nominal_unit=K  temperature_nominal_value=1
  + : PMIOPort  Side=Left
  - : PMIOPort  Port=2  Side=Left
  Current : Outport
  wires:
  Current sensor/1(i) -> Scope/1, Current/1
  q/1 -> Actuator/1(q)
  connections:
  Diode/LConn1 -- Electrical Reference/LConn1 -- -/RConn1 -- r_b_2/RConn1
  Solver Configuration/RConn1 -- +/RConn1 -- N-Channel MOSFET/RConn1
  r_b_1/LConn1 -- r_f/RConn1
  Current sensor/LConn1 -- Diode/RConn1 -- N-Channel MOSFET/RConn2 -- Actuator/RConn2
  l_f/LConn1 -- r_f/LConn1
  l_f/RConn1 -- r_b_2/LConn1
  Current sensor/RConn1 -- r_b_1/RConn1
  Actuator/RConn1 -- N-Channel MOSFET/LConn1

== system AutomotiveEMS_2017b/Alternator/Stator Inductance (abc reference) ==
  i_f : Inport
  Mux : Mux  Inputs=3
  statorInductance : MATLAB Function  TreatAsAtomicUnit=on
  l_abc : Outport
  wires:
  statorInductance/1(l_s) -> Mux/3, Mux/1, Mux/2
  i_f/1 -> statorInductance/1(i_f)
  Mux/1 -> l_abc/1

== system AutomotiveEMS_2017b/Three-phase diode rectifier/D1 ==
  Diode : elec_lib/Semiconductor Devices/Diode  ModelType=1  Vf=0.6 V  Ron=0.3 Ohm  Goff=1e-8 S  Rz=0.3 Ohm  Vz=50 V  C_PWL=5 pF  prmExp=1  I12=[.0137, .545] A  V12=[.6, .7] V  I1=0.0137 A  V1=0.6 V  IS=1e-12 A  ec=1  RS=0.01 Ohm  Tmeas=25 degC  BV=inf V  C_param=1  CJ0=5 pF  VJ=1 V  Mgrad=0.5  Vvec=[.1, 10, 100] V  Cvec=[3.5, 1, .4] pF  FC=0.5  Q_param=1  Irrm=-7.15 A  iF=4 A  didt=-750 A/us  trr=115 ns  TT=50 ns  tau=100 ns  T_param=1  IS_T2=1.25e-7 A  I1_T2=0.245 A  V1_T2=0.5 V  Tmeas2=125 degC  EG_param=1  EG=1.11 eV  XTI_param=1  XTI=3  dBVdT=0 V/K  Tdevice=25 degC  i_capacitor_specify=off  i_capacitor_priority=High  i_capacitor=0 A  i_capacitor_nominal_specify=off  i_capacitor_nominal_unit=A  i_capacitor_nominal_value=1  v_capacitor_specify=off  v_capacitor_priority=None  v_capacitor=0 V  v_capacitor_nominal_specify=off  v_capacitor_nominal_unit=V  v_capacitor_nominal_value=1  Rth=[0, 10] K/W  thermal_mass_parameterization=1  thermal_mass=[0, 1] J/K  thermal_time_constant=[0, 10] s  thermal_mass_initial_temperatures=[25, 25] degC
      settings: SourceProductName=Simscape Electronics  SourceProductBaseCode=SN
  current sensor : Subsystem
  m : Scope  NumInputPorts=2
  voltage sensor : Subsystem
  - : PMIOPort  Side=Right
  + : PMIOPort  Port=2  Side=Left
  wires:
  voltage sensor/1(v) -> m/1
  current sensor/1(i) -> m/2
  connections:
  Diode/RConn1 -- -/RConn1 -- voltage sensor/LConn1
  voltage sensor/RConn1 -- Diode/LConn1 -- current sensor/RConn1
  +/RConn1 -- current sensor/LConn1

== system AutomotiveEMS_2017b/Three-phase diode rectifier/D2 ==
  Diode : elec_lib/Semiconductor Devices/Diode  ModelType=1  Vf=0.6 V  Ron=0.3 Ohm  Goff=1e-8 S  Rz=0.3 Ohm  Vz=50 V  C_PWL=5 pF  prmExp=1  I12=[.0137, .545] A  V12=[.6, .7] V  I1=0.0137 A  V1=0.6 V  IS=1e-12 A  ec=1  RS=0.01 Ohm  Tmeas=25 degC  BV=inf V  C_param=1  CJ0=5 pF  VJ=1 V  Mgrad=0.5  Vvec=[.1, 10, 100] V  Cvec=[3.5, 1, .4] pF  FC=0.5  Q_param=1  Irrm=-7.15 A  iF=4 A  didt=-750 A/us  trr=115 ns  TT=50 ns  tau=100 ns  T_param=1  IS_T2=1.25e-7 A  I1_T2=0.245 A  V1_T2=0.5 V  Tmeas2=125 degC  EG_param=1  EG=1.11 eV  XTI_param=1  XTI=3  dBVdT=0 V/K  Tdevice=25 degC  i_capacitor_specify=off  i_capacitor_priority=High  i_capacitor=0 A  i_capacitor_nominal_specify=off  i_capacitor_nominal_unit=A  i_capacitor_nominal_value=1  v_capacitor_specify=off  v_capacitor_priority=None  v_capacitor=0 V  v_capacitor_nominal_specify=off  v_capacitor_nominal_unit=V  v_capacitor_nominal_value=1  Rth=[0, 10] K/W  thermal_mass_parameterization=1  thermal_mass=[0, 1] J/K  thermal_time_constant=[0, 10] s  thermal_mass_initial_temperatures=[25, 25] degC
      settings: SourceProductName=Simscape Electronics  SourceProductBaseCode=SN
  current sensor : Subsystem
  m : Scope  NumInputPorts=2
  voltage sensor : Subsystem
  - : PMIOPort  Side=Right
  + : PMIOPort  Port=2  Side=Left
  wires:
  voltage sensor/1(v) -> m/1
  current sensor/1(i) -> m/2
  connections:
  Diode/RConn1 -- -/RConn1 -- voltage sensor/LConn1
  voltage sensor/RConn1 -- Diode/LConn1 -- current sensor/RConn1
  +/RConn1 -- current sensor/LConn1

== system AutomotiveEMS_2017b/Three-phase diode rectifier/D3 ==
  Diode : elec_lib/Semiconductor Devices/Diode  ModelType=1  Vf=0.6 V  Ron=0.3 Ohm  Goff=1e-8 S  Rz=0.3 Ohm  Vz=50 V  C_PWL=5 pF  prmExp=1  I12=[.0137, .545] A  V12=[.6, .7] V  I1=0.0137 A  V1=0.6 V  IS=1e-12 A  ec=1  RS=0.01 Ohm  Tmeas=25 degC  BV=inf V  C_param=1  CJ0=5 pF  VJ=1 V  Mgrad=0.5  Vvec=[.1, 10, 100] V  Cvec=[3.5, 1, .4] pF  FC=0.5  Q_param=1  Irrm=-7.15 A  iF=4 A  didt=-750 A/us  trr=115 ns  TT=50 ns  tau=100 ns  T_param=1  IS_T2=1.25e-7 A  I1_T2=0.245 A  V1_T2=0.5 V  Tmeas2=125 degC  EG_param=1  EG=1.11 eV  XTI_param=1  XTI=3  dBVdT=0 V/K  Tdevice=25 degC  i_capacitor_specify=off  i_capacitor_priority=High  i_capacitor=0 A  i_capacitor_nominal_specify=off  i_capacitor_nominal_unit=A  i_capacitor_nominal_value=1  v_capacitor_specify=off  v_capacitor_priority=None  v_capacitor=0 V  v_capacitor_nominal_specify=off  v_capacitor_nominal_unit=V  v_capacitor_nominal_value=1  Rth=[0, 10] K/W  thermal_mass_parameterization=1  thermal_mass=[0, 1] J/K  thermal_time_constant=[0, 10] s  thermal_mass_initial_temperatures=[25, 25] degC
      settings: SourceProductName=Simscape Electronics  SourceProductBaseCode=SN
  current sensor : Subsystem
  m : Scope  NumInputPorts=2
  voltage sensor : Subsystem
  - : PMIOPort  Side=Right
  + : PMIOPort  Port=2  Side=Left
  wires:
  voltage sensor/1(v) -> m/1
  current sensor/1(i) -> m/2
  connections:
  Diode/RConn1 -- -/RConn1 -- voltage sensor/LConn1
  voltage sensor/RConn1 -- Diode/LConn1 -- current sensor/RConn1
  +/RConn1 -- current sensor/LConn1

== system AutomotiveEMS_2017b/Three-phase diode rectifier/D4 ==
  Diode : elec_lib/Semiconductor Devices/Diode  ModelType=1  Vf=0.6 V  Ron=0.3 Ohm  Goff=1e-8 S  Rz=0.3 Ohm  Vz=50 V  C_PWL=5 pF  prmExp=1  I12=[.0137, .545] A  V12=[.6, .7] V  I1=0.0137 A  V1=0.6 V  IS=1e-12 A  ec=1  RS=0.01 Ohm  Tmeas=25 degC  BV=inf V  C_param=1  CJ0=5 pF  VJ=1 V  Mgrad=0.5  Vvec=[.1, 10, 100] V  Cvec=[3.5, 1, .4] pF  FC=0.5  Q_param=1  Irrm=-7.15 A  iF=4 A  didt=-750 A/us  trr=115 ns  TT=50 ns  tau=100 ns  T_param=1  IS_T2=1.25e-7 A  I1_T2=0.245 A  V1_T2=0.5 V  Tmeas2=125 degC  EG_param=1  EG=1.11 eV  XTI_param=1  XTI=3  dBVdT=0 V/K  Tdevice=25 degC  i_capacitor_specify=off  i_capacitor_priority=High  i_capacitor=0 A  i_capacitor_nominal_specify=off  i_capacitor_nominal_unit=A  i_capacitor_nominal_value=1  v_capacitor_specify=off  v_capacitor_priority=None  v_capacitor=0 V  v_capacitor_nominal_specify=off  v_capacitor_nominal_unit=V  v_capacitor_nominal_value=1  Rth=[0, 10] K/W  thermal_mass_parameterization=1  thermal_mass=[0, 1] J/K  thermal_time_constant=[0, 10] s  thermal_mass_initial_temperatures=[25, 25] degC
      settings: SourceProductName=Simscape Electronics  SourceProductBaseCode=SN
  current sensor : Subsystem
  m : Scope  NumInputPorts=2
  voltage sensor : Subsystem
  - : PMIOPort  Side=Right
  + : PMIOPort  Port=2  Side=Left
  wires:
  voltage sensor/1(v) -> m/1
  current sensor/1(i) -> m/2
  connections:
  Diode/RConn1 -- -/RConn1 -- voltage sensor/LConn1
  voltage sensor/RConn1 -- Diode/LConn1 -- current sensor/RConn1
  +/RConn1 -- current sensor/LConn1

== system AutomotiveEMS_2017b/Three-phase diode rectifier/D5 ==
  Diode : elec_lib/Semiconductor Devices/Diode  ModelType=1  Vf=0.6 V  Ron=0.3 Ohm  Goff=1e-8 S  Rz=0.3 Ohm  Vz=50 V  C_PWL=5 pF  prmExp=1  I12=[.0137, .545] A  V12=[.6, .7] V  I1=0.0137 A  V1=0.6 V  IS=1e-12 A  ec=1  RS=0.01 Ohm  Tmeas=25 degC  BV=inf V  C_param=1  CJ0=5 pF  VJ=1 V  Mgrad=0.5  Vvec=[.1, 10, 100] V  Cvec=[3.5, 1, .4] pF  FC=0.5  Q_param=1  Irrm=-7.15 A  iF=4 A  didt=-750 A/us  trr=115 ns  TT=50 ns  tau=100 ns  T_param=1  IS_T2=1.25e-7 A  I1_T2=0.245 A  V1_T2=0.5 V  Tmeas2=125 degC  EG_param=1  EG=1.11 eV  XTI_param=1  XTI=3  dBVdT=0 V/K  Tdevice=25 degC  i_capacitor_specify=off  i_capacitor_priority=High  i_capacitor=0 A  i_capacitor_nominal_specify=off  i_capacitor_nominal_unit=A  i_capacitor_nominal_value=1  v_capacitor_specify=off  v_capacitor_priority=None  v_capacitor=0 V  v_capacitor_nominal_specify=off  v_capacitor_nominal_unit=V  v_capacitor_nominal_value=1  Rth=[0, 10] K/W  thermal_mass_parameterization=1  thermal_mass=[0, 1] J/K  thermal_time_constant=[0, 10] s  thermal_mass_initial_temperatures=[25, 25] degC
      settings: SourceProductName=Simscape Electronics  SourceProductBaseCode=SN
  current sensor : Subsystem
  m : Scope  NumInputPorts=2
  voltage sensor : Subsystem
  - : PMIOPort  Side=Right
  + : PMIOPort  Port=2  Side=Left
  wires:
  voltage sensor/1(v) -> m/1
  current sensor/1(i) -> m/2
  connections:
  Diode/RConn1 -- -/RConn1 -- voltage sensor/LConn1
  voltage sensor/RConn1 -- Diode/LConn1 -- current sensor/RConn1
  +/RConn1 -- current sensor/LConn1

== system AutomotiveEMS_2017b/Three-phase diode rectifier/D6 ==
  Diode : elec_lib/Semiconductor Devices/Diode  ModelType=1  Vf=0.6 V  Ron=0.3 Ohm  Goff=1e-8 S  Rz=0.3 Ohm  Vz=50 V  C_PWL=5 pF  prmExp=1  I12=[.0137, .545] A  V12=[.6, .7] V  I1=0.0137 A  V1=0.6 V  IS=1e-12 A  ec=1  RS=0.01 Ohm  Tmeas=25 degC  BV=inf V  C_param=1  CJ0=5 pF  VJ=1 V  Mgrad=0.5  Vvec=[.1, 10, 100] V  Cvec=[3.5, 1, .4] pF  FC=0.5  Q_param=1  Irrm=-7.15 A  iF=4 A  didt=-750 A/us  trr=115 ns  TT=50 ns  tau=100 ns  T_param=1  IS_T2=1.25e-7 A  I1_T2=0.245 A  V1_T2=0.5 V  Tmeas2=125 degC  EG_param=1  EG=1.11 eV  XTI_param=1  XTI=3  dBVdT=0 V/K  Tdevice=25 degC  i_capacitor_specify=off  i_capacitor_priority=High  i_capacitor=0 A  i_capacitor_nominal_specify=off  i_capacitor_nominal_unit=A  i_capacitor_nominal_value=1  v_capacitor_specify=off  v_capacitor_priority=None  v_capacitor=0 V  v_capacitor_nominal_specify=off  v_capacitor_nominal_unit=V  v_capacitor_nominal_value=1  Rth=[0, 10] K/W  thermal_mass_parameterization=1  thermal_mass=[0, 1] J/K  thermal_time_constant=[0, 10] s  thermal_mass_initial_temperatures=[25, 25] degC
      settings: SourceProductName=Simscape Electronics  SourceProductBaseCode=SN
  current sensor : Subsystem
  m : Scope  NumInputPorts=2
  voltage sensor : Subsystem
  - : PMIOPort  Side=Right
  + : PMIOPort  Port=2  Side=Left
  wires:
  voltage sensor/1(v) -> m/1
  current sensor/1(i) -> m/2
  connections:
  Diode/RConn1 -- -/RConn1 -- voltage sensor/LConn1
  voltage sensor/RConn1 -- Diode/LConn1 -- current sensor/RConn1
  +/RConn1 -- current sensor/LConn1

== system AutomotiveEMS_2017b/Three-phase diode rectifier/i_a sensor ==
  Current Sensor : fl_lib/Electrical/Electrical Sensors/Current Sensor
  PS-Simulink Converter : nesl_utility/PS-Simulink Converter  PhysicalDomain=network_engine_domain  SubClassName=ps_output  LeftPortType=input  RightPortType=output  PseudoPeriodic=off  Frequencies=[]  Unit=1  AffineConversion=off
  + : PMIOPort  Side=Left
  - : PMIOPort  Port=2  Side=Right
  i : Outport
  wires:
  PS-Simulink Converter/1 -> i/1
  connections:
  Current Sensor/RConn2 -- -/RConn1
  Current Sensor/LConn1 -- +/RConn1
  PS-Simulink Converter/LConn1 -- Current Sensor/RConn1

== system AutomotiveEMS_2017b/Three-phase diode rectifier/v_o sensor ==
  PS-Simulink Converter : nesl_utility/PS-Simulink Converter  PhysicalDomain=network_engine_domain  SubClassName=ps_output  LeftPortType=input  RightPortType=output  PseudoPeriodic=off  Frequencies=[]  Unit=1  AffineConversion=off
  Voltage Sensor : fl_lib/Electrical/Electrical Sensors/Voltage Sensor
  + : PMIOPort  Side=Left
  - : PMIOPort  Port=2  Side=Right
  v : Outport
  wires:
  PS-Simulink Converter/1 -> v/1
  connections:
  Voltage Sensor/LConn1 -- +/RConn1
  -/RConn1 -- Voltage Sensor/RConn2
  Voltage Sensor/RConn1 -- PS-Simulink Converter/LConn1

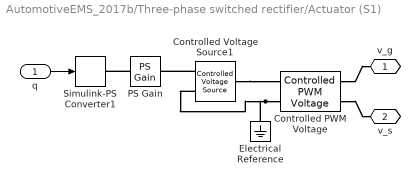
== system AutomotiveEMS_2017b/Three-phase switched rectifier/Actuator (S1) ==
  q : Inport
  Controlled PWM Voltage : elec_lib/Actuators & Drivers/Drivers/Controlled PWM Voltage  F=rectifier.control.pwm.f_s Hz  TD=0 s  pulse_width_offset=0 s  pulse_min=0 s  Vmin=rectifier.control.pwm.v_clear V  Vmax=rectifier.control.pwm.v_set V  Vm=rectifier.control.pwm.v_out V  pwm_or_av=1  event_type=1  sample_time=1e-6 s  u_min=0  u_max=1
      settings: SourceProductName=Simscape Electronics  SourceProductBaseCode=SN
  Controlled Voltage Source1 : fl_lib/Electrical/Electrical Sources/Controlled Voltage Source
  Electrical Reference : fl_lib/Electrical/Electrical Elements/Electrical Reference
  PS Gain : fl_lib/Physical Signals/Functions/PS Gain  gain=rectifier.control.pwm.v_set
  Simulink-PS Converter1 : nesl_utility/Simulink-PS Converter  PhysicalDomain=network_engine_domain  SubClassName=ps_input  LeftPortType=input  RightPortType=output  PseudoPeriodic=off  Frequencies=[]  NoiseDistribution=none  NoiseParameters=[]  Unit=1  AffineConversion=off  FilteringAndDerivatives=provide  SimscapeFilterOrder=1  InputFilterTimeConstant=0.001  UdotUserProvided=0
  v_g : PMIOPort  Side=Right
  v_s : PMIOPort  Port=2  Side=Right
  wires:
  q/1 -> Simulink-PS Converter1/1
  connections:
  Controlled Voltage Source1/LConn1 -- Controlled PWM Voltage/LConn1
  Controlled PWM Voltage/RConn2 -- v_s/RConn1
  Controlled PWM Voltage/RConn1 -- v_g/RConn1
  PS Gain/LConn1 -- Simulink-PS Converter1/RConn1
  Controlled PWM Voltage/LConn2 -- Controlled Voltage Source1/RConn2 -- Electrical Reference/LConn1
  Controlled Voltage Source1/RConn1 -- PS Gain/RConn1

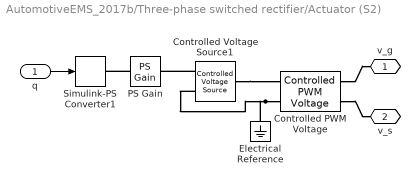
== system AutomotiveEMS_2017b/Three-phase switched rectifier/Actuator (S2) ==
  q : Inport
  Controlled PWM Voltage : elec_lib/Actuators & Drivers/Drivers/Controlled PWM Voltage  F=rectifier.control.pwm.f_s Hz  TD=0 s  pulse_width_offset=0 s  pulse_min=0 s  Vmin=rectifier.control.pwm.v_clear V  Vmax=rectifier.control.pwm.v_set V  Vm=rectifier.control.pwm.v_out V  pwm_or_av=1  event_type=1  sample_time=1e-6 s  u_min=0  u_max=1
      settings: SourceProductName=Simscape Electronics  SourceProductBaseCode=SN
  Controlled Voltage Source1 : fl_lib/Electrical/Electrical Sources/Controlled Voltage Source
  Electrical Reference : fl_lib/Electrical/Electrical Elements/Electrical Reference
  PS Gain : fl_lib/Physical Signals/Functions/PS Gain  gain=rectifier.control.pwm.v_set
  Simulink-PS Converter1 : nesl_utility/Simulink-PS Converter  PhysicalDomain=network_engine_domain  SubClassName=ps_input  LeftPortType=input  RightPortType=output  PseudoPeriodic=off  Frequencies=[]  NoiseDistribution=none  NoiseParameters=[]  Unit=1  AffineConversion=off  FilteringAndDerivatives=provide  SimscapeFilterOrder=1  InputFilterTimeConstant=0.001  UdotUserProvided=0
  v_g : PMIOPort  Side=Right
  v_s : PMIOPort  Port=2  Side=Right
  wires:
  q/1 -> Simulink-PS Converter1/1
  connections:
  Controlled Voltage Source1/LConn1 -- Controlled PWM Voltage/LConn1
  Controlled PWM Voltage/RConn2 -- v_s/RConn1
  Controlled PWM Voltage/RConn1 -- v_g/RConn1
  PS Gain/LConn1 -- Simulink-PS Converter1/RConn1
  Controlled PWM Voltage/LConn2 -- Controlled Voltage Source1/RConn2 -- Electrical Reference/LConn1
  Controlled Voltage Source1/RConn1 -- PS Gain/RConn1
